simulink library "Cross_Product_3D_lib"  (Simulink 6.6)
libraries: simulink x1
settings Model: Creator=cbuttril  LastModifiedBy=cbuttril

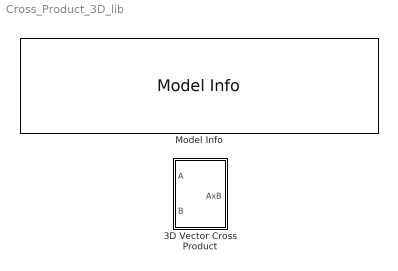
== system Cross_Product_3D_lib ==
  3D Vector Cross Product : Subsystem
  Model Info : simulink/Model-Wide Utilities/Model Info  SystemSampleTime=-1  InitialBlockCM=None  BlockCM=None  Frame=on  DisplayStringWithTags=|  HorizontalTextAlignment=Center  LeftAlignmentValue=0.5  SourceBlockDiagram=Cross_Product_3D_lib  TagMaxNumber=20
      | Developed using Matlab Release 2007a
      | 
      | SVN:%<ModelVersion>
      | Last modifed by %<LastModifiedBy> on %<LastModificationDate>

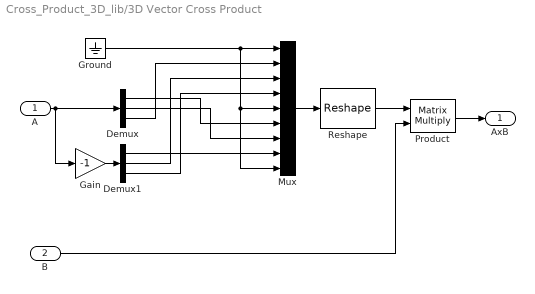
== system Cross_Product_3D_lib/3D Vector Cross Product ==
  A : Inport
  B : Inport  Port=2
  Demux : Demux  Outputs=3
  Demux1 : Demux  Outputs=3
  Gain : Gain  Gain=-1  SaturateOnIntegerOverflow=on
  Ground : Ground
  Mux : Mux  Inputs=9
  Product : Product  Multiplication=Matrix(*)  SaturateOnIntegerOverflow=on
  Reshape : Reshape  OutputDimensionality=Customize  OutputDimensions=[3,3]
  AxB : Outport
  wires:
  B/1 -> Product/2
  Reshape/1 -> Product/1
  Mux/1 -> Reshape/1
  Demux1/1 -> Mux/8
  Demux/2 -> Mux/7
  Demux/1 -> Mux/6
  Demux1/3 -> Mux/4
  Demux1/2 -> Mux/3
  Demux/3 -> Mux/2
  Gain/1 -> Demux1/1
  Ground/1 -> Mux/9, Mux/5, Mux/1
  Product/1 -> AxB/1
  A/1 -> Gain/1, Demux/1
